simulink library "Room_Floor_Heating"  (R2013b)
settings: Solver=ode45  StartTime=0.0  StopTime=10.0  RelTol=1e-3
libraries: carnot x17
settings Model: Creator=lena.frank  LastModifiedBy=drhf

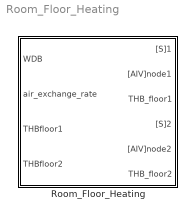
== system Room_Floor_Heating ==
  Room_Floor_Heating : Subsystem  mask(room){t0=20, temp_neighbour=20}
      mask prompts: t0 "start temperature of rooms in °C"; temp_neighbour "temperature of rooms above and below in °C"
      mask help:
      | The block models of a heat transfer characteristic of two neighbour rooms.
      | Use "look under mask" to set up the models parameters (initial conditions,
      | floors and wall characteristics...)
      mask init:
      | AIV_neighbour = [0 temp_neighbour temp_neighbour 0 0 0 0 0 0];
      | zonefloordist2grnd = 0;
      mask Help: web(fullfile(path_carnot('help'),'Room_Floor_Heating.html'),'-helpbrowser')
      mask Display: plot(0,0,100,100,[30,30,60,60,30],[20,50,50,20,20],[47,47,56,56,47],[40,30,30,40,40],[42,42,34,34],[20,40,40,20],[62,45,28],[48,70,48])

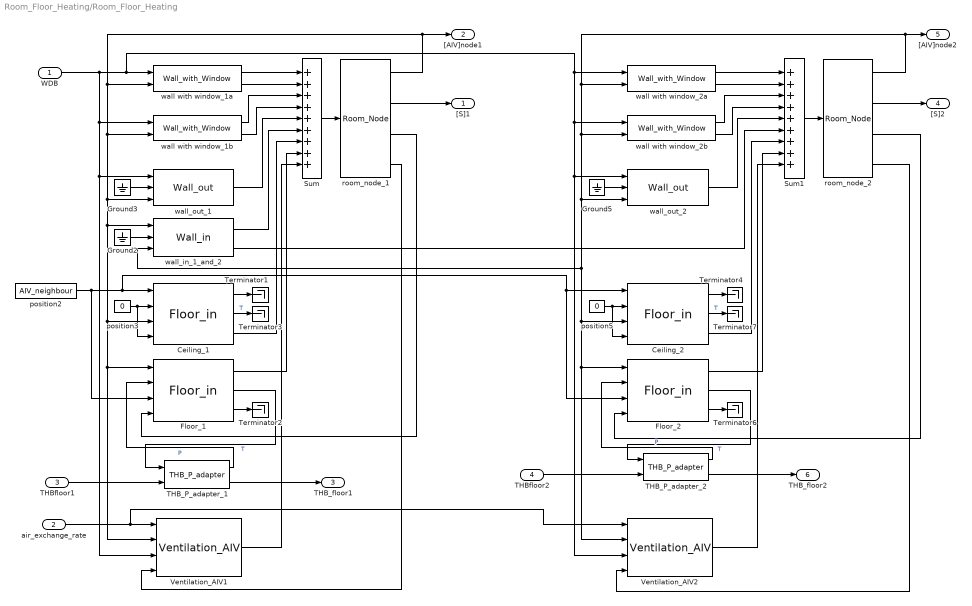
== system Room_Floor_Heating/Room_Floor_Heating ==
  WDB : Inport
  air_exchange_rate : Inport  Port=2
  THBfloor1 : Inport  Port=3
  THBfloor2 : Inport  Port=4
  Ceiling_1 : carnot/Load/Houses/wall_floor/Floor_in  wallsize=[5 5]  t0=20  d=[0.015 0.38 0.02]  cond=[1.4 0.79 0.7]  cwall=[0.28 0.28 0.28]*3600  rho=[2000 1800 1400]  misc=[.65 .65]  dactive=-1  tau=1000*3600
  Ceiling_2 : carnot/Load/Houses/wall_floor/Floor_in  wallsize=[5 5]  t0=20  d=[0.015 0.38 0.02]  cond=[1.4 0.79 0.7]  cwall=[0.28 0.28 0.28]*3600  rho=[2000 1800 1400]  misc=[.65 .65]  dactive=-1  tau=1000*3600
  Floor_1 : carnot/Load/Houses/wall_floor/Floor_in  wallsize=[5 5]  t0=20  d=[0.015 0.38 0.02]  cond=[1.4 0.79 0.7]  cwall=[0.28 0.28 0.28]*3600  rho=[2000 1800 1400]  misc=[.65 .65]  dactive=0.02  tau=1000*3600
  Floor_2 : carnot/Load/Houses/wall_floor/Floor_in  wallsize=[5 5]  t0=20  d=[0.015 0.38 0.02]  cond=[1.4 0.79 0.7]  cwall=[0.28 0.28 0.28]*3600  rho=[2000 1800 1400]  misc=[.65 .65]  dactive=0.02  tau=1000*3600
  Ground2 : Ground
  Ground3 : Ground
  Ground5 : Ground
  Sum : Sum  Inputs=9  SaturateOnIntegerOverflow=on  InputSameDT=on  OutDataTypeStr=Inherit: Same as first input
  Sum1 : Sum  Inputs=9  SaturateOnIntegerOverflow=on  InputSameDT=on  OutDataTypeStr=Inherit: Same as first input
  THB_P_adapter_1 : carnot/Load/Houses/ventilation_heating/THB_P_adapter  mass=1  ua=800*5*5/0.2*0.022*3.1415  t0=20
  THB_P_adapter_2 : carnot/Load/Houses/ventilation_heating/THB_P_adapter  mass=1  ua=800*5*5/0.2*0.022*3.1415  t0=20
  Terminator{1..4,6..7} (6 alike) : Terminator
  Ventilation_AIV1 : carnot/Source/Ventilation/Ventilation_AIV  co2=400
  Ventilation_AIV2 : carnot/Source/Ventilation/Ventilation_AIV  co2=400
  position2 : Constant  Value=AIV_neighbour
  position3 : Constant  Value=0
  position5 : Constant  Value=0
  room_node_1 : carnot/Load/Houses/room_node/Room_Node  zoneairvolume=5*5*2.5  zoneheight=2.5  zonestartTEMP=20  zonestartWATER=55  timeconst=100  heatperfect=natural  lookuptime=[0 24]*3600  lookupvalue=[20 20]  AirPressure=101300
  room_node_2 : carnot/Load/Houses/room_node/Room_Node  zoneairvolume=5*5*2.5  zoneheight=2.5  zonestartTEMP=20  zonestartWATER=55  timeconst=100  heatperfect=natural  lookuptime=[0 24]*3600  lookupvalue=[20 20]  AirPressure=101300
  wall with window_1a : carnot/Load/Houses/wall_floor/Wall_with_Window  wallsize=[2.5 5]  windowsize=[1 2]  frame=0.1  pos=90  t0=20  tau=1000*3600  g=0.7
  wall with window_1b : carnot/Load/Houses/wall_floor/Wall_with_Window  wallsize=[2.5 5]  windowsize=[1 2]  frame=0.1  pos=0  t0=20  tau=1000*3600  g=0.7
  wall with window_2a : carnot/Load/Houses/wall_floor/Wall_with_Window  wallsize=[2.5 5]  windowsize=[1 2]  frame=0.1  pos=-90  t0=20  tau=1000*3600  g=0.7
  wall with window_2b : carnot/Load/Houses/wall_floor/Wall_with_Window  wallsize=[2.5 5]  windowsize=[1 2]  frame=0.1  pos=0  t0=20  tau=1000*3600  g=0.7
  wall_in_1_and_2 : carnot/Load/Houses/wall_floor/Wall_in  wallsize=[2.5 5]  d=[0.015 0.38 0.02]  cond=[1.4 0.79 0.7]  cwall=[0.28 0.28 0.28]*3600  rho=[2000 1800 1400]  emission_in=.96  dactive=-1  t0=20  tau=1000*3600
  wall_out_1 : carnot/Load/Houses/wall_floor/Wall_out  wallsize=[2.5 5]  pos=180  t0=20  d=[0.1 0.38]  cond=[0.04 0.79]  cwall=[0.28 0.28]*3600  rho=[900 1800]  reflectground=0.2  abs_emiss=[0.65 0.97 0.96]  tau=1000*3600  dactive=-1
  wall_out_2 : carnot/Load/Houses/wall_floor/Wall_out  wallsize=[2.5 5]  pos=180  t0=20  d=[0.1 0.38]  cond=[0.04 0.79]  cwall=[0.28 0.28]*3600  rho=[900 1800]  reflectground=0.2  abs_emiss=[0.65 0.97 0.96]  tau=1000*3600  dactive=-1
  "[S]1" : Outport
  "[AIV]node1" : Outport  Port=2
  THB_floor1 : Outport  Port=3
  "[S]2" : Outport  Port=4
  "[AIV]node2" : Outport  Port=5
  THB_floor2 : Outport  Port=6
  wires:
  Sum1/1 -> room_node_2/1
  Sum/1 -> room_node_1/1
  room_node_2/1 -> "[AIV]node2"/1, wall with window_2a/2, wall with window_2b/2, wall_in_1_and_2/3, Ceiling_2/3, Ventilation_AIV2/2, Floor_2/1, wall_out_2/3
  room_node_1/1 -> "[AIV]node1"/1, wall_out_1/3, Ventilation_AIV1/2, Floor_1/1, Ceiling_1/3, wall_in_1_and_2/1, wall with window_1b/2, wall with window_1a/2
  air_exchange_rate/1 -> Ventilation_AIV1/1, Ventilation_AIV2/1
  wall_in_1_and_2/2 -> Sum1/6
  Ground5/1 -> wall_out_2/2
  room_node_2/3 -> Floor_2/4
  room_node_2/4 -> Ventilation_AIV2/4
  THB_P_adapter_2/2 -> THB_floor2/1
  THB_P_adapter_2/1 -> Floor_2/2  "P"
  Floor_2/2 -> THB_P_adapter_2/1  "T"
  THBfloor2/1 -> THB_P_adapter_2/2
  Ventilation_AIV2/1 -> Sum1/9
  Ceiling_2/3 -> Sum1/7
  Floor_2/1 -> Sum1/8
  position5/1 -> Ceiling_2/2, Ceiling_2/4
  Floor_2/3 -> Terminator6/1
  Ceiling_2/2 -> Terminator7/1  "T"
  Ceiling_2/1 -> Terminator4/1
  room_node_2/2 -> "[S]2"/1
  wall with window_2b/2 -> Sum1/4
  wall_out_2/1 -> Sum1/5
  wall with window_2b/1 -> Sum1/3
  wall with window_2a/2 -> Sum1/2
  wall with window_2a/1 -> Sum1/1
  position2/1 -> Floor_2/3, Ceiling_2/1, Ceiling_1/1, Floor_1/3
  Ground3/1 -> wall_out_1/2
  Ground2/1 -> wall_in_1_and_2/2
  room_node_1/3 -> Floor_1/4
  room_node_1/4 -> Ventilation_AIV1/4
  THB_P_adapter_1/2 -> THB_floor1/1
  THB_P_adapter_1/1 -> Floor_1/2  "P"
  Floor_1/2 -> THB_P_adapter_1/1  "T"
  THBfloor1/1 -> THB_P_adapter_1/2
  Ventilation_AIV1/1 -> Sum/9
  Ceiling_1/3 -> Sum/7
  Floor_1/1 -> Sum/8
  position3/1 -> Ceiling_1/4, Ceiling_1/2
  Floor_1/3 -> Terminator2/1
  Ceiling_1/2 -> Terminator3/1  "T"
  Ceiling_1/1 -> Terminator1/1
  room_node_1/2 -> "[S]1"/1
  wall with window_1b/2 -> Sum/4
  wall_out_1/1 -> Sum/5
  wall with window_1b/1 -> Sum/3
  wall with window_1a/2 -> Sum/2
  wall with window_1a/1 -> Sum/1
  WDB/1 -> wall with window_2a/1, wall with window_2b/1, Ventilation_AIV2/3, wall_out_2/1, wall with window_1a/1, Ventilation_AIV1/3, wall_out_1/1, wall with window_1b/1
  wall_in_1_and_2/1 -> Sum/6
